simulink model "OML58_Cores"  (R2021b)
settings: Solver=ode4  StartTime=0.0  StopTime=inf  FixedStep=Ts  RelTol=1e-3  EnableMultiTasking=on
PostLoadFcn:
  | Ts = 50e-6;
InitFcn:
  | Ts = 50e-6;
undefined symbols (not defined in the file): I, Left, Right, type, V
libraries: spsSeriesRLCBranchLib x24, spsThreePhaseSeriesRLCLoadLib x12, spsThreePhaseSeriesRLCBranchLib x12, spsThreePhaseBreakerLib x12, artemis x10, spsGroundLib x8, rtlab x6, LafaeLib x6, spsThreePhaseTransformerTwoWindingsLib x5, spsThreePhaseVIMeasurementLib x5, spsPower3phInstantaneousLib x3, spsThreePhaseSourceLib x1
(part 3 of 3)

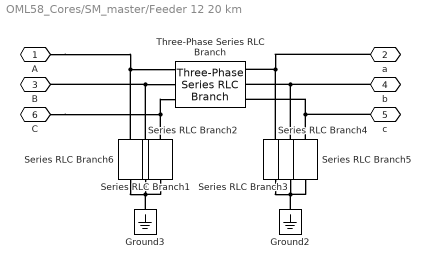
== system OML58_Cores/SM_master/Feeder 12 20 km ==
  Ground2 : spsGroundLib/Ground  LConnTagsString=a
  Ground3 : spsGroundLib/Ground  LConnTagsString=a
  Series RLC Branch{1..6} (6 alike) : spsSeriesRLCBranchLib/Series RLC Branch  LConnTagsString=__new0  RConnTagsString=__new0  BranchType=C  Resistance=1  Inductance=1e-3  SetiL0=off  InitialCurrent=0  Capacitance=l*0.495e-6/2  Setx0=off  InitialVoltage=0  Measurements=None
  Three-Phase Series RLC Branch : spsThreePhaseSeriesRLCBranchLib/Three-Phase Series RLC Branch  LConnTagsString=A|B|C  RConnTagsString=A|B|C  BranchType=RL  Resistance=l*0.0991  Inductance=l*0.602e-3  Capacitance=1e-6  Measurements=None
  A : PMIOPort  Side=Left
  a : PMIOPort  Port=2  Side=Right
  B : PMIOPort  Port=3  Side=Left
  b : PMIOPort  Port=4  Side=Right
  c : PMIOPort  Port=5  Side=Right
  C : PMIOPort  Port=6  Side=Left
  connections:
  Ground2/LConn1 -- Series RLC Branch5/RConn1 -- Series RLC Branch4/RConn1 -- Series RLC Branch3/RConn1
  Series RLC Branch2/LConn1 -- C/RConn1 -- Three-Phase Series RLC Branch/LConn3
  Ground3/LConn1 -- Series RLC Branch2/RConn1 -- Series RLC Branch1/RConn1 -- Series RLC Branch6/RConn1
  Series RLC Branch3/LConn1 -- a/RConn1 -- Three-Phase Series RLC Branch/RConn1
  Series RLC Branch6/LConn1 -- A/RConn1 -- Three-Phase Series RLC Branch/LConn1
  Series RLC Branch4/LConn1 -- b/RConn1 -- Three-Phase Series RLC Branch/RConn2
  Series RLC Branch5/LConn1 -- c/RConn1 -- Three-Phase Series RLC Branch/RConn3
  Series RLC Branch1/LConn1 -- B/RConn1 -- Three-Phase Series RLC Branch/LConn2

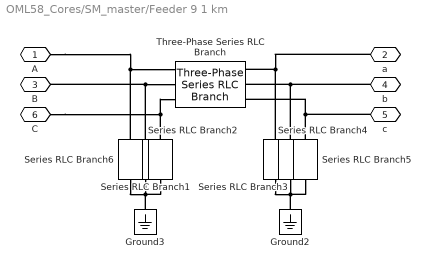
== system OML58_Cores/SM_master/Feeder 9 1 km ==
  Ground2 : spsGroundLib/Ground  LConnTagsString=a
  Ground3 : spsGroundLib/Ground  LConnTagsString=a
  Series RLC Branch{1..6} (6 alike) : spsSeriesRLCBranchLib/Series RLC Branch  LConnTagsString=__new0  RConnTagsString=__new0  BranchType=C  Resistance=1  Inductance=1e-3  SetiL0=off  InitialCurrent=0  Capacitance=l*0.495e-6/2  Setx0=off  InitialVoltage=0  Measurements=None
  Three-Phase Series RLC Branch : spsThreePhaseSeriesRLCBranchLib/Three-Phase Series RLC Branch  LConnTagsString=A|B|C  RConnTagsString=A|B|C  BranchType=RL  Resistance=l*0.0991  Inductance=l*0.602e-3  Capacitance=1e-6  Measurements=None
  A : PMIOPort  Side=Left
  a : PMIOPort  Port=2  Side=Right
  B : PMIOPort  Port=3  Side=Left
  b : PMIOPort  Port=4  Side=Right
  c : PMIOPort  Port=5  Side=Right
  C : PMIOPort  Port=6  Side=Left
  connections:
  Ground2/LConn1 -- Series RLC Branch5/RConn1 -- Series RLC Branch4/RConn1 -- Series RLC Branch3/RConn1
  Series RLC Branch2/LConn1 -- C/RConn1 -- Three-Phase Series RLC Branch/LConn3
  Ground3/LConn1 -- Series RLC Branch2/RConn1 -- Series RLC Branch1/RConn1 -- Series RLC Branch6/RConn1
  Series RLC Branch3/LConn1 -- a/RConn1 -- Three-Phase Series RLC Branch/RConn1
  Series RLC Branch6/LConn1 -- A/RConn1 -- Three-Phase Series RLC Branch/LConn1
  Series RLC Branch4/LConn1 -- b/RConn1 -- Three-Phase Series RLC Branch/RConn2
  Series RLC Branch5/LConn1 -- c/RConn1 -- Three-Phase Series RLC Branch/RConn3
  Series RLC Branch1/LConn1 -- B/RConn1 -- Three-Phase Series RLC Branch/LConn2

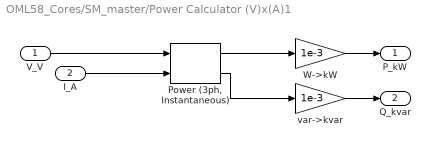
== system OML58_Cores/SM_master/Power Calculator (V)x(A)1 ==
  V_V : Inport
  I_A : Inport  Port=2
  "Power (3ph, Instantaneous)" : spsPower3phInstantaneousLib/Power (3ph, Instantaneous)
  W->kW : Gain  Gain=1e-3
  var->kvar : Gain  Gain=1e-3
  P_kW : Outport
  Q_kvar : Outport  Port=2
  wires:
  V_V/1 -> "Power (3ph, Instantaneous)"/1
  I_A/1 -> "Power (3ph, Instantaneous)"/2
  "Power (3ph, Instantaneous)"/1 -> W->kW/1
  "Power (3ph, Instantaneous)"/2 -> var->kvar/1
  W->kW/1 -> P_kW/1
  var->kvar/1 -> Q_kvar/1

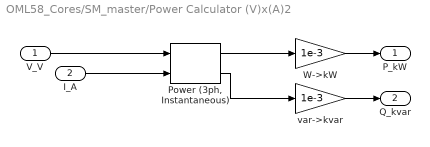
== system OML58_Cores/SM_master/Power Calculator (V)x(A)2 ==
  V_V : Inport
  I_A : Inport  Port=2
  "Power (3ph, Instantaneous)" : spsPower3phInstantaneousLib/Power (3ph, Instantaneous)
  W->kW : Gain  Gain=1e-3
  var->kvar : Gain  Gain=1e-3
  P_kW : Outport
  Q_kvar : Outport  Port=2
  wires:
  V_V/1 -> "Power (3ph, Instantaneous)"/1
  I_A/1 -> "Power (3ph, Instantaneous)"/2
  "Power (3ph, Instantaneous)"/1 -> W->kW/1
  "Power (3ph, Instantaneous)"/2 -> var->kvar/1
  W->kW/1 -> P_kW/1
  var->kvar/1 -> Q_kvar/1

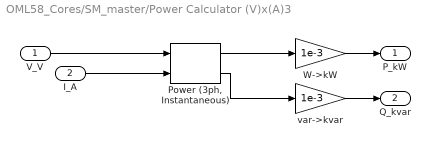
== system OML58_Cores/SM_master/Power Calculator (V)x(A)3 ==
  V_V : Inport
  I_A : Inport  Port=2
  "Power (3ph, Instantaneous)" : spsPower3phInstantaneousLib/Power (3ph, Instantaneous)
  W->kW : Gain  Gain=1e-3
  var->kvar : Gain  Gain=1e-3
  P_kW : Outport
  Q_kvar : Outport  Port=2
  wires:
  V_V/1 -> "Power (3ph, Instantaneous)"/1
  I_A/1 -> "Power (3ph, Instantaneous)"/2
  "Power (3ph, Instantaneous)"/1 -> W->kW/1
  "Power (3ph, Instantaneous)"/2 -> var->kvar/1
  W->kW/1 -> P_kW/1
  var->kvar/1 -> Q_kvar/1

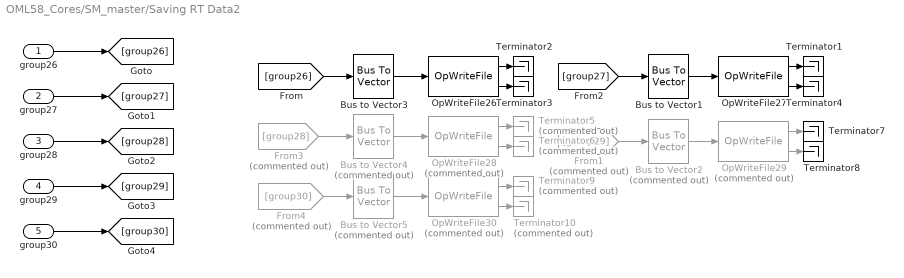
== system OML58_Cores/SM_master/Saving RT Data2 ==
  group26 : Inport
  group27 : Inport  Port=2
  group28 : Inport  Port=3
  group29 : Inport  Port=4
  group30 : Inport  Port=5
  Bus to Vector1 : BusToVector
  Bus to Vector2 : BusToVector  Commented=on
  Bus to Vector3 : BusToVector
  Bus to Vector4 : BusToVector  Commented=on
  Bus to Vector5 : BusToVector  Commented=on
  From1 : From  Commented=on  GotoTag=group29
  From3 : From  Commented=on  GotoTag=group28
  From4 : From  Commented=on  GotoTag=group30
  OpWriteFile26 : rtlab/DataLogging/OpWriteFile  Static_File=on  varname=BESS_m  Filename=BESS_m.mat  rtpath='./'  nrtpath='.\'  Acq_Group=26  file_size=(nls26+1)*8*(ld26/Ts)*1.5  write_offline=on  Sim_Mode=off  Nb_Samples=ld26/Ts  Buffer_size=(ld26/Ts)*8*(1+nls26)
      settings: SourceProductName=RT-LAB  Decimation=Decimation26
  OpWriteFile27 : rtlab/DataLogging/OpWriteFile  Static_File=on  varname=Load_L  Filename=Load_L.mat  rtpath='./'  nrtpath='.\'  Acq_Group=27  file_size=(nls27+1)*8*(ld27/Ts)*1.5  write_offline=on  Sim_Mode=off  Nb_Samples=ld27/Ts  Buffer_size=(ld26/Ts)*8*(1+nls26)
      settings: SourceProductName=RT-LAB  Decimation=Decimation27
  OpWriteFile28 : rtlab/DataLogging/OpWriteFile  Commented=on  Static_File=on  varname=Meas_Q  Filename=Meas_Q.mat  rtpath='./'  nrtpath='.\'  Acq_Group=28  file_size=(nls28+1)*8*(ld28/Ts)*1.5  write_offline=on  Sim_Mode=off  Nb_Samples=ld28/Ts  Buffer_size=(ld28/Ts)*8*(1+nls28)
      settings: SourceProductName=RT-LAB  Decimation=Decimation28
  OpWriteFile29 : rtlab/DataLogging/OpWriteFile  Commented=on  Static_File=on  varname=P_Loads  Filename=P_Loads.mat  rtpath='./'  nrtpath='.\'  Acq_Group=29  file_size=(nls29+1)*8*(ld29/Ts)*1.5  write_offline=on  Sim_Mode=off  Nb_Samples=ld29/Ts  Buffer_size=(ld29/Ts)*8*(1+nls29)
      settings: SourceProductName=RT-LAB  Decimation=Decimation29
  OpWriteFile30 : rtlab/DataLogging/OpWriteFile  Commented=on  Static_File=on  varname=Q_Loads  Filename=Q_Loads.mat  rtpath='./'  nrtpath='.\'  Acq_Group=30  file_size=(nls30+1)*8*(ld30/Ts)*1.5  write_offline=on  Sim_Mode=off  Nb_Samples=ld30/Ts  Buffer_size=(ld30/Ts)*8*(1+nls30)
      settings: SourceProductName=RT-LAB  Decimation=Decimation30
  Terminator{1..4,7..8} (6 alike) : Terminator
  Terminator{5..6,9..10} (4 alike) : Terminator  Commented=on
  wires:
  OpWriteFile28/2 -> Terminator6/1
  OpWriteFile27/1 -> Terminator1/1
  OpWriteFile26/2 -> Terminator3/1
  OpWriteFile26/1 -> Terminator2/1
  OpWriteFile30/1 -> Terminator9/1
  OpWriteFile27/2 -> Terminator4/1
  OpWriteFile29/2 -> Terminator8/1
  OpWriteFile30/2 -> Terminator10/1
  OpWriteFile29/1 -> Terminator7/1
  OpWriteFile28/1 -> Terminator5/1
  group26/1 -> [group26]
  group27/1 -> [group27]
  group28/1 -> [group28]
  group29/1 -> [group29]
  group30/1 -> [group30]
  [group27] -> Bus to Vector1/1
  Bus to Vector1/1 -> OpWriteFile27/1
  From1/1 -> Bus to Vector2/1
  Bus to Vector2/1 -> OpWriteFile29/1
  [group26] -> Bus to Vector3/1
  Bus to Vector3/1 -> OpWriteFile26/1
  From3/1 -> Bus to Vector4/1
  Bus to Vector4/1 -> OpWriteFile28/1
  From4/1 -> Bus to Vector5/1
  Bus to Vector5/1 -> OpWriteFile30/1
